simulink model "BME_project_Adaptive"  (R2020a)
settings: Solver=VariableStepAuto  StartTime=0.0  StopTime=400  RelTol=1e-3
settings Model: Creator=sunda  LastModifiedBy=sunda

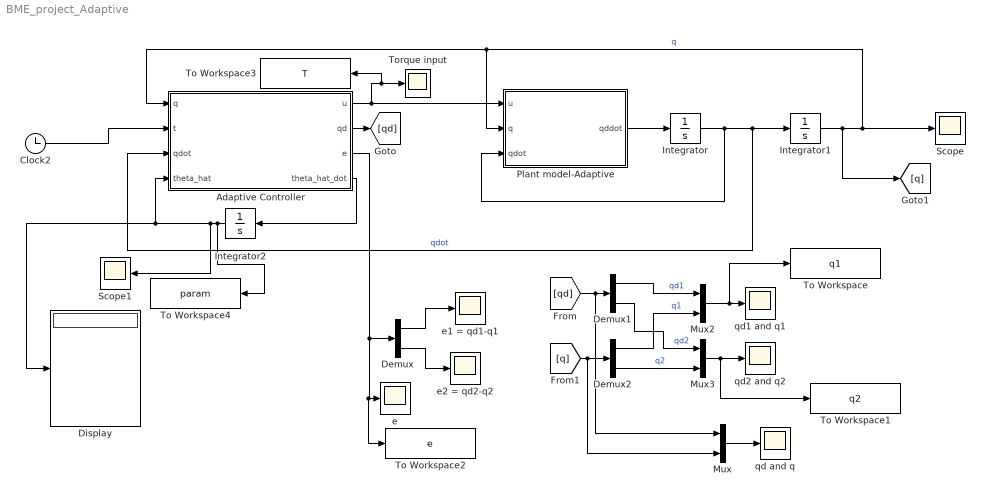
== system BME_project_Adaptive ==
  " Torque input" : Scope
  Adaptive Controller : MATLAB Function  TreatAsAtomicUnit=on
  Clock2 : Clock
  Demux : Demux  Outputs=2
  Demux1 : Demux  Outputs=2
  Demux2 : Demux  Outputs=2
  Display : Display
      settings: Decimation=5
  Integrator : Integrator  InitialCondition=zeros(2,1)
  Integrator1 : Integrator  InitialCondition=zeros(2,1)
  Integrator2 : Integrator  InitialCondition=[0;0.2;0.2;1;1]
  Mux : Mux  Inputs=2
  Mux2 : Mux  Inputs=2
  Mux3 : Mux  Inputs=2
  Plant model-Adaptive : MATLAB Function  TreatAsAtomicUnit=on
  Scope : Scope
  Scope1 : Scope
  To Workspace : ToWorkspace  VariableName=q1  SaveFormat=Timeseries  SampleTime=-1
  To Workspace1 : ToWorkspace  VariableName=q2  SaveFormat=Timeseries  SampleTime=-1
  To Workspace2 : ToWorkspace  VariableName=e  SaveFormat=Timeseries  SampleTime=-1
  To Workspace3 : ToWorkspace  VariableName=T  SaveFormat=Timeseries  SampleTime=-1
  To Workspace4 : ToWorkspace  VariableName=param  SaveFormat=Timeseries  SampleTime=-1
  e : Scope
  e1 = qd1-q1 : Scope
  e2 = qd2-q2 : Scope
  qd and q : Scope
  qd1 and q1 : Scope
  qd2 and q2 : Scope
  wires:
  Integrator1/1 -> [q], Plant model-Adaptive/2(q), Adaptive Controller/1(q), Scope/1  "q"
  Integrator/1 -> Integrator1/1, Adaptive Controller/3(qdot), Plant model-Adaptive/3(qdot)  "qdot"
  Plant model-Adaptive/1(qddot) -> Integrator/1
  Clock2/1 -> Adaptive Controller/2(t)
  Adaptive Controller/4(theta_hat_dot) -> Integrator2/1
  Integrator2/1 -> To Workspace4/1, Scope1/1, Display/1, Adaptive Controller/4(theta_hat)
  [q] -> Mux/2, Demux2/1
  Mux2/1 -> To Workspace/1, qd1 and q1/1
  [qd] -> Mux/1, Demux1/1
  Mux/1 -> qd and q/1
  Mux3/1 -> To Workspace1/1, qd2 and q2/1
  Demux2/1 -> Mux2/2  "q1"
  Demux2/2 -> Mux3/2  "q2"
  Demux1/1 -> Mux2/1  "qd1"
  Demux1/2 -> Mux3/1  "qd2"
  Demux/1 -> e1 = qd1-q1/1
  Adaptive Controller/3(e) -> Demux/1, To Workspace2/1, e/1
  Demux/2 -> e2 = qd2-q2/1
  Adaptive Controller/2(qd) -> [qd]
  Adaptive Controller/1(u) -> Plant model-Adaptive/1(u), To Workspace3/1, " Torque input"/1

== matlab function BME_project_Adaptive/Adaptive Controller ==
  data: q input; u output; t input; qdot input; qd output; e output; theta_hat input; theta_hat_dot output
%% Adaptive controller

function [u,qd,e,theta_hat_dot] = fcn(q,t,qdot,theta_hat)

q1 = q(1);
q2 = q(2);

q1dot =qdot(1);
q2dot = qdot(2);
  
qd = [cos(t) cos(2*t)]';
qd_dot = [-sin(t) -2* sin(2*t)]';
qd_ddot = [-cos(t) -4*cos(2*t)]';

e = qd-q;
e_dot =qd_dot - qdot;


% Gain values

alpha = 2; 
K = 15*eye(2);
gamma = 0.5*eye(5);
r = e_dot + alpha *e;
 
Y = [qd_ddot(1)+alpha*e_dot(1)   qd_ddot(2)+alpha*e_dot(2)      2*cos(q2)*(qd_ddot(1)+alpha*e_dot(1))+cos(q2)*qd_ddot(2)+alpha*e_dot(2)-sin(q2)*q2dot*(qd_dot(1)+alpha*e(1))-sin(q2)*(q1dot+q2dot)*(qd_dot(2)+alpha*e(2))   q1dot   0;...
            0          qd_ddot(1)+alpha*e_dot(1)+qd_ddot(2)+alpha*e_dot(2)      cos(q2)*(qd_ddot(1)+alpha*e_dot(1))+sin(q2)*q1dot*(qd_dot(1)+alpha*e(1))    0   q2dot];

theta_hat_dot = gamma\Y'*r;
%%% Control law - Adaptive

u = Y*theta_hat+K*r;

end

== matlab function BME_project_Adaptive/Plant model-Adaptive ==
  data: u input; q input; qdot input; qddot output
%% Robot Plant model - Adaptive
function qddot = fcn(u,q,qdot)

q1 = q(1);
q2 = q(2);

q1dot =qdot(1);
q2dot = qdot(2);

p1 = 3.473; %%% kg.m^2
p2 = 0.196; %%% kg.m^2
p3 = 0.242; %%% kg.m^2

fd1 = 5.3; %%% N.m.sec
fd2 = 1.1; %%% N.m.sec
%%% Disturbance
% Td1 = 0.3;   %%% N.m
% Td2 = 0.3;   %%% N.m
%%% No disturbance
Td1 = 0.0;   %%% N.m
Td2 = 0.0;   %%% N.m
%%% Inertia matrix M(q)
M =[p1+2*p3*cos(q2)     p2 + p3*cos(q2);...
    p2 + p3* cos(q2)        p2];

%%% Centripetal and Coriollis term V(q,qdot)

Vm = [-p3*sin(q2)*q2dot     -p3*sin(q2)*(q1dot +q2dot);...
     p3* sin(q2)*q1dot                  0];
 
%% Damping/ friction term 

Fd = [fd1   0;
      0     fd2];
  
%% Disturbance:

Td = [Td1 Td2]';
%%% Robot dynamics of a Two - link Robot

qddot = inv(M)*(u - Vm*qdot -Fd*qdot - Td);

end
